simulink library "Gait_Selector"  (R2024a)
settings: Solver=VariableStepAuto  StartTime=0.0  StopTime=10.0  RelTol=1e-3
undefined symbols (not defined in the file): Length_torso, sampleTime, transferFunVal, Width_torso
libraries: simulink_extras x12, stand_still_Gait x1, trot_Gait x1, turn_left_Gait x1, turn_right_Gait x1, walk_back_Gait x1, walk_Gait x1, walk_left_Gait x1, walk_right_Gait x1
(part 1 of 2)
settings Model: Creator=renre  LastModifiedBy=leona

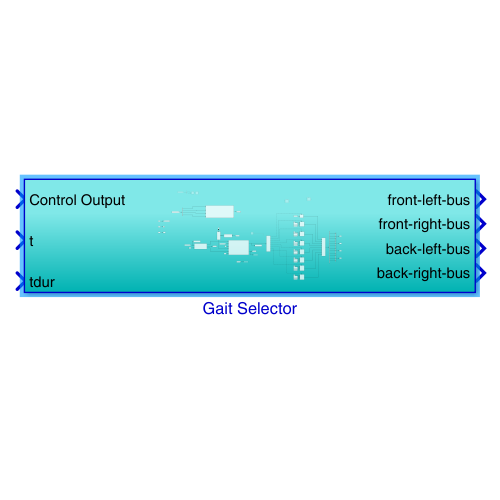
[thumbnail: Simulink's stored preview of the top-level diagram]
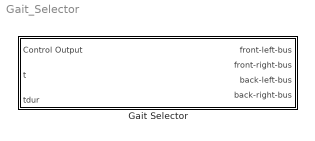
== system Gait_Selector ==
  Gait Selector : Subsystem

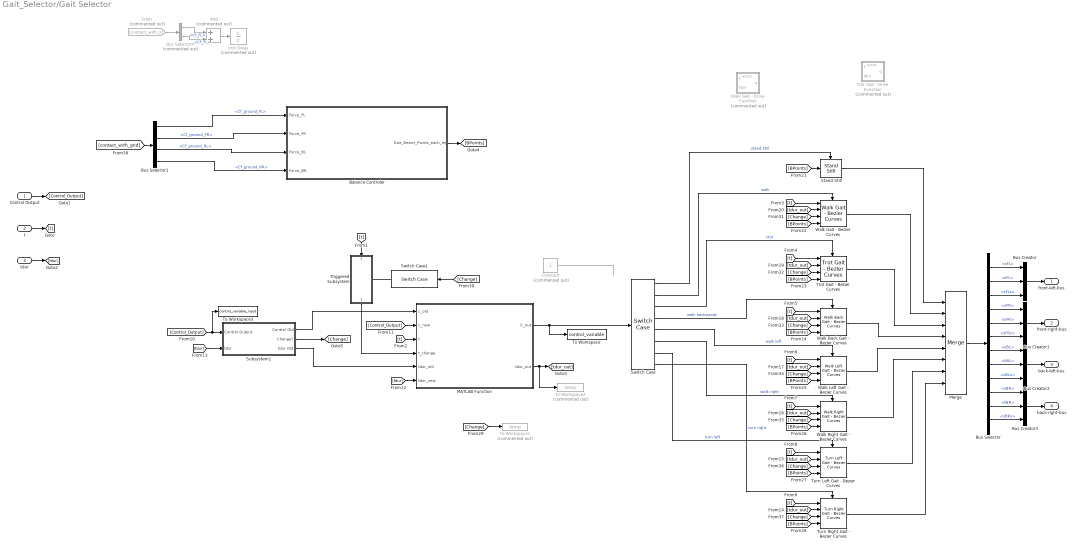
== system Gait_Selector/Gait Selector ==
  Control Output : Inport
  t : Inport  Port=2
  tdur : Inport  Port=3
  Add : Sum  Commented=on
  Balance Controler : Subsystem
  Bus Creator{,1..3} (4 alike) : BusCreator  Inputs=3
  Bus Selector : BusSelector  OutputSignals=sFL,kFL,sFLs,sFR,kFR,sFRs,sBL,kBL,sBLs,sBR,kBR,sBRs
  Bus Selector1 : BusSelector  OutputSignals=Cf_ground_FL,Cf_ground_FR,Cf_ground_RL,Cf_ground_RR
  Bus Selector4 : BusSelector  Commented=on  OutputSignals=Wall.Cf_FL,Slope.Cf_FL
  Constant : Constant  Commented=on
  From : From  Commented=on  GotoTag=contact_with_x  TagVisibility=global
  MATLAB Function : MATLAB Function  TreatAsAtomicUnit=on
  Merge : Merge  Inputs=8
  Stand Still : stand_still_Gait/Stand Still  SystemSampleTime=-1  VariantActivationTime=update diagram  AllowFlexibleInterface=on  Latency=0  AutoFrameSizeCalculation=off
  Subsystem1 : Subsystem
  Switch Case : SwitchCase  CaseConditions={0,1,2,3,4,5,6,7}  ShowDefaultCase=off
  Switch Case1 : SwitchCase  ShowDefaultCase=off
  To Workspace : ToWorkspace  VariableName=control_variable  SaveFormat=Structure With Time  SampleTime=-1
  To Workspace1 : ToWorkspace  Commented=on  VariableName=temp  SaveFormat=Structure With Time  SampleTime=-1
  To Workspace2 : ToWorkspace  Commented=on  VariableName=temp  SaveFormat=Structure With Time  SampleTime=-1
  To Workspace3 : ToWorkspace  VariableName=control_variable_input  SaveFormat=Structure With Time  SampleTime=-1
  Triggered Subsystem : Subsystem  TreatAsAtomicUnit=on
  Trot Gait - Bezier Curves : trot_Gait/Trot Gait - Bezier Curves  SystemSampleTime=-1  VariantActivationTime=update diagram  AllowFlexibleInterface=on  Latency=0  AutoFrameSizeCalculation=off
  Trot Gait - Drive Function : Subsystem  Commented=on  mask{uMin=30-20, uMax=30+10, lMin=-50, lMax=-35}
      mask prompts: uMin "Min Angle Hip"; uMax "Max Angle Hip"; lMin "Min Angle Knee"; lMax "Max Angle Knee"
  Turn Left Gait - Bezier Curves : turn_left_Gait/Turn Left Gait - Bezier Curves  SystemSampleTime=-1  VariantActivationTime=update diagram  AllowFlexibleInterface=on  Latency=0  AutoFrameSizeCalculation=off
  Turn Right Gait - Bezier Curves : turn_right_Gait/Turn Right Gait - Bezier Curves  SystemSampleTime=-1  VariantActivationTime=update diagram  AllowFlexibleInterface=on  Latency=0  AutoFrameSizeCalculation=off
  Unit Delay : UnitDelay  Commented=on  SampleTime=-1  HasFrameUpgradeWarning=on
  Walk Back Gait - Bezier Curves : walk_back_Gait/Walk Back Gait - Bezier Curves  SystemSampleTime=-1  VariantActivationTime=update diagram  AllowFlexibleInterface=on  Latency=0  AutoFrameSizeCalculation=off
  Walk Gait - Bezier Curves : walk_Gait/Walk Gait - Bezier Curves  SystemSampleTime=-1  VariantActivationTime=update diagram  AllowFlexibleInterface=on  Latency=0  AutoFrameSizeCalculation=off
  Walk Gait - Drive Function : Subsystem  Commented=on  mask{uMin=30-20, uMax=30+10, lMin=-50, lMax=-35}
      mask prompts: uMin "Min Angle Hip"; uMax "Max Angle Hip"; lMin "Min Angle Knee"; lMax "Max Angle Knee"
  Walk Left Gait - Bezier Curves : walk_left_Gait/Walk Left Gait - Bezier Curves  SystemSampleTime=-1  VariantActivationTime=update diagram  AllowFlexibleInterface=on  Latency=0  AutoFrameSizeCalculation=off
  Walk Right Gait - Bezier Curves : walk_right_Gait/Walk Right Gait - Bezier Curves  SystemSampleTime=-1  VariantActivationTime=update diagram  AllowFlexibleInterface=on  Latency=0  AutoFrameSizeCalculation=off
  front-left-bus : Outport
  front-right-bus : Outport  Port=2
  back-left-bus : Outport  Port=3
  back-right-bus : Outport  Port=4
  wires:
  Control Output/1 -> [Control_Output]
  t/1 -> [t]
  Bus Creator/1 -> front-left-bus/1
  Bus Creator1/1 -> front-right-bus/1
  Bus Creator2/1 -> back-left-bus/1
  Bus Creator3/1 -> back-right-bus/1
  Switch Case/2 -> Walk Gait - Bezier Curves/Action  "walk"
  Switch Case/3 -> Trot Gait - Bezier Curves/Action  "trot"
  Switch Case/5 -> Walk Left Gait - Bezier Curves/Action  "walk left"
  Switch Case/6 -> Walk Right Gait - Bezier Curves/Action  "walk right"
  Switch Case/7 -> Turn Left Gait - Bezier Curves/Action  "turn left"
  Switch Case/8 -> Turn Right Gait - Bezier Curves/Action  "turn right"
  MATLAB Function/2(tdur_out) -> To Workspace2/1, [tdur_out]
  Merge/1 -> Bus Selector/1
  Walk Gait - Bezier Curves/1 -> Merge/2
  Bus Selector/1 -> Bus Creator/1  "<sFL>"
  Bus Selector/2 -> Bus Creator/2  "<kFL>"
  Bus Selector/6 -> Bus Creator1/3  "<sFRs>"
  Bus Selector/5 -> Bus Creator1/2  "<kFR>"
  Bus Selector/7 -> Bus Creator2/1  "<sBL>"
  Bus Selector/8 -> Bus Creator2/2  "<kBL>"
  Bus Selector/12 -> Bus Creator3/3  "<sBRs>"
  Trot Gait - Bezier Curves/1 -> Merge/3
  Bus Selector/11 -> Bus Creator3/2  "<kBR>"
  Walk Left Gait - Bezier Curves/1 -> Merge/5
  Bus Selector/3 -> Bus Creator/3  "<sFLs>"
  Bus Selector/4 -> Bus Creator1/1  "<sFR>"
  Bus Selector/10 -> Bus Creator3/1  "<sBR>"
  Bus Selector/9 -> Bus Creator2/3  "<sBLs>"
  Walk Right Gait - Bezier Curves/1 -> Merge/6
  Turn Left Gait - Bezier Curves/1 -> Merge/7
  Turn Right Gait - Bezier Curves/1 -> Merge/8
  Switch Case/4 -> Walk Back Gait - Bezier Curves/Action  "walk backwards"
  Walk Back Gait - Bezier Curves/1 -> Merge/4
  Stand Still/1 -> Merge/1
  Switch Case/1 -> Stand Still/Action  "stand still"
  Subsystem1/2(Change?) -> [Change]
  MATLAB Function/1(C_out) -> Switch Case/1, To Workspace/1
  Subsystem1/1(Control Old) -> MATLAB Function/1(c_old)
  tdur/1 -> [tdur]
  Subsystem1/3(tdur Old) -> MATLAB Function/5(tdur_old)
  Triggered Subsystem/1(activationTime) -> MATLAB Function/4(t_change)
  Switch Case1/1 -> Triggered Subsystem/Action
  Constant/1 -> ?
  Balance Controler/1(Gait_Bezier_Points_each_leg) -> [BPoints]
  Add/1 -> Unit Delay/1
  From/1 -> Bus Selector4/1
  Bus Selector4/1 -> Add/1  "<Cf_FL>"
  Bus Selector4/2 -> Add/2  "<Cf_FL>"
  [t] -> Triggered Subsystem/1(t)
  [t] -> MATLAB Function/3(t)
  [t] -> Walk Gait - Bezier Curves/1
  [t] -> Trot Gait - Bezier Curves/1
  [t] -> Walk Back Gait - Bezier Curves/1
  [t] -> Walk Left Gait - Bezier Curves/1
  [t] -> Walk Right Gait - Bezier Curves/1
  [t] -> Turn Left Gait - Bezier Curves/1
  [t] -> Turn Right Gait - Bezier Curves/1
  [Control_Output] -> To Workspace3/1, Subsystem1/1(Control Output)
  [Control_Output] -> MATLAB Function/2(c_new)
  [tdur] -> Subsystem1/2(tdur)
  [tdur] -> MATLAB Function/6(tdur_new)
  [tdur_out] -> Turn Right Gait - Bezier Curves/2
  [tdur_out] -> Turn Left Gait - Bezier Curves/2
  [tdur_out] -> Walk Right Gait - Bezier Curves/2
  [tdur_out] -> Walk Left Gait - Bezier Curves/2
  [tdur_out] -> Walk Back Gait - Bezier Curves/2
  [tdur_out] -> Trot Gait - Bezier Curves/2
  [tdur_out] -> Walk Gait - Bezier Curves/2
  [BPoints] -> Stand Still/1
  [BPoints] -> Walk Gait - Bezier Curves/4
  [BPoints] -> Trot Gait - Bezier Curves/4
  [BPoints] -> Walk Back Gait - Bezier Curves/4
  [BPoints] -> Walk Left Gait - Bezier Curves/4
  [BPoints] -> Walk Right Gait - Bezier Curves/4
  [BPoints] -> Turn Left Gait - Bezier Curves/4
  [BPoints] -> Turn Right Gait - Bezier Curves/4
  [Change] -> To Workspace1/1
  [Change] -> Switch Case1/1
  [Change] -> Walk Gait - Bezier Curves/3
  [Change] -> Trot Gait - Bezier Curves/3
  [Change] -> Walk Back Gait - Bezier Curves/3
  [Change] -> Walk Left Gait - Bezier Curves/3
  [Change] -> Walk Right Gait - Bezier Curves/3
  [Change] -> Turn Left Gait - Bezier Curves/3
  [Change] -> Turn Right Gait - Bezier Curves/3
  [contact_with_grid] -> Bus Selector1/1
  Bus Selector1/3 -> Balance Controler/3(Force_BL)  "<Cf_ground_RL>"
  Bus Selector1/4 -> Balance Controler/4(Force_BR)  "<Cf_ground_RR>"
  Bus Selector1/1 -> Balance Controler/1(Force_FL)  "<Cf_ground_FL>"
  Bus Selector1/2 -> Balance Controler/2(Force_FR)  "<Cf_ground_FR>"

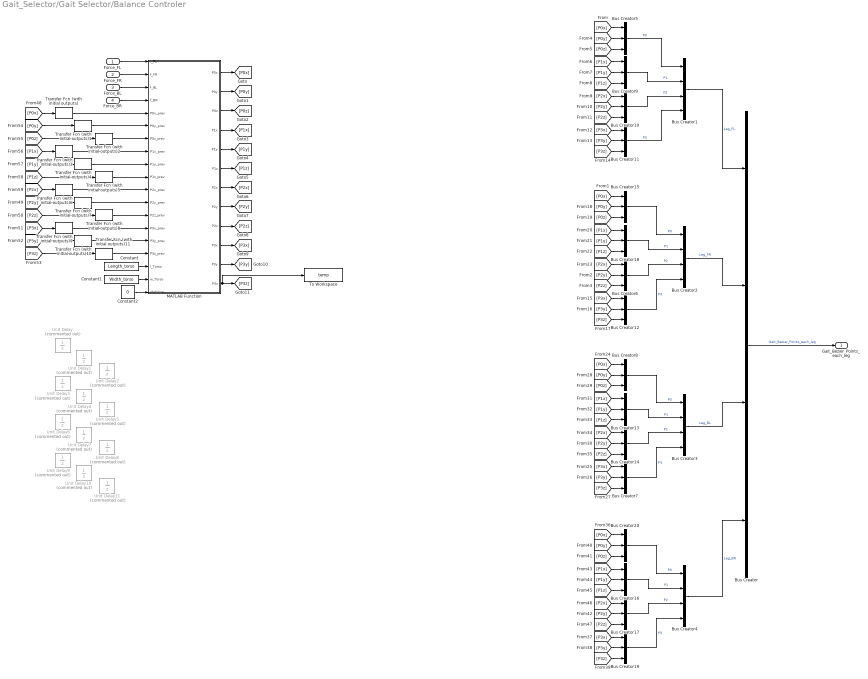
== system Gait_Selector/Gait Selector/Balance Controler ==
  Force_FL : Inport
  Force_FR : Inport  Port=2
  Force_BL : Inport  Port=3
  Force_BR : Inport  Port=4
  Bus Creator{,1..4} (5 alike) : BusCreator  Inputs=4
  Bus Creator{5..20} (16 alike) : BusCreator  Inputs=3
  Constant : Constant  Value=Length_torso
  Constant1 : Constant  Value=Width_torso
  Constant2 : Constant  Value=0
  MATLAB Function : MATLAB Function  TreatAsAtomicUnit=on
  To Workspace : ToWorkspace  VariableName=temp  SaveFormat=Structure With Time  SampleTime=-1
  Transfer Fcn (with initial outputs) : simulink_extras/Additional Linear/Transfer Fcn (with initial outputs)  N=[1]  D=transferFunVal  Y0=-0.02  U0=0
  Transfer Fcn (with initial outputs)1 : simulink_extras/Additional Linear/Transfer Fcn (with initial outputs)  N=[1]  D=transferFunVal  Y0=-0.02  U0=0
  Transfer Fcn (with initial outputs)10 : simulink_extras/Additional Linear/Transfer Fcn (with initial outputs)  N=[1]  D=transferFunVal  Y0=0.02  U0=0
  Transfer Fcn (with initial outputs)11 : simulink_extras/Additional Linear/Transfer Fcn (with initial outputs)  N=[1]  D=transferFunVal  Y0=-0.08  U0=0
  Transfer Fcn (with initial outputs)2 : simulink_extras/Additional Linear/Transfer Fcn (with initial outputs)  N=[1]  D=transferFunVal  Y0=-0.08  U0=0
  Transfer Fcn (with initial outputs)3 : simulink_extras/Additional Linear/Transfer Fcn (with initial outputs)  N=[1]  D=transferFunVal  Y0=-0.035  U0=0
  Transfer Fcn (with initial outputs)4 : simulink_extras/Additional Linear/Transfer Fcn (with initial outputs)  N=[1]  D=transferFunVal  Y0=-0.035  U0=0
  Transfer Fcn (with initial outputs)5 : simulink_extras/Additional Linear/Transfer Fcn (with initial outputs)  N=[1]  D=transferFunVal  Y0=-0.075  U0=0
  Transfer Fcn (with initial outputs)6 : simulink_extras/Additional Linear/Transfer Fcn (with initial outputs)  N=[1]  D=transferFunVal  Y0=0.01  U0=0
  Transfer Fcn (with initial outputs)7 : simulink_extras/Additional Linear/Transfer Fcn (with initial outputs)  N=[1]  D=transferFunVal  Y0=0.01  U0=0
  Transfer Fcn (with initial outputs)8 : simulink_extras/Additional Linear/Transfer Fcn (with initial outputs)  N=[1]  D=transferFunVal  Y0=-0.075  U0=0
  Transfer Fcn (with initial outputs)9 : simulink_extras/Additional Linear/Transfer Fcn (with initial outputs)  N=[1]  D=transferFunVal  Y0=0.02  U0=0
  Unit Delay : UnitDelay  Commented=on  InitialCondition=-0.02  SampleTime=sampleTime  HasFrameUpgradeWarning=on
  Unit Delay1 : UnitDelay  Commented=on  InitialCondition=-0.02  SampleTime=sampleTime  HasFrameUpgradeWarning=on
  Unit Delay10 : UnitDelay  Commented=on  InitialCondition=0.02  SampleTime=sampleTime  HasFrameUpgradeWarning=on
  Unit Delay11 : UnitDelay  Commented=on  InitialCondition=-0.08  SampleTime=sampleTime  HasFrameUpgradeWarning=on
  Unit Delay2 : UnitDelay  Commented=on  InitialCondition=-0.08  SampleTime=sampleTime  HasFrameUpgradeWarning=on
  Unit Delay3 : UnitDelay  Commented=on  InitialCondition=-0.035  SampleTime=sampleTime  HasFrameUpgradeWarning=on
  Unit Delay4 : UnitDelay  Commented=on  InitialCondition=-0.035  SampleTime=sampleTime  HasFrameUpgradeWarning=on
  Unit Delay5 : UnitDelay  Commented=on  InitialCondition=-0.06  SampleTime=sampleTime  HasFrameUpgradeWarning=on
  Unit Delay6 : UnitDelay  Commented=on  InitialCondition=0.01  SampleTime=sampleTime  HasFrameUpgradeWarning=on
  Unit Delay7 : UnitDelay  Commented=on  InitialCondition=0.01  SampleTime=sampleTime  HasFrameUpgradeWarning=on
  Unit Delay8 : UnitDelay  Commented=on  InitialCondition=-0.075  SampleTime=sampleTime  HasFrameUpgradeWarning=on
  Unit Delay9 : UnitDelay  Commented=on  InitialCondition=0.02  SampleTime=sampleTime  HasFrameUpgradeWarning=on
  Gait_Bezier_Points_each_leg : Outport
  wires:
  Bus Creator1/1 -> Bus Creator/1  "Leg_FL"
  Bus Creator2/1 -> Bus Creator/2  "Leg_FR"
  Bus Creator3/1 -> Bus Creator/3  "Leg_BL"
  Bus Creator4/1 -> Bus Creator/4  "Leg_BR"
  Bus Creator/1 -> Gait_Bezier_Points_each_leg/1  "Gait_Bezier_Points_each_leg"
  Bus Creator5/1 -> Bus Creator1/1  "P0"
  Bus Creator9/1 -> Bus Creator1/2  "P1"
  Bus Creator10/1 -> Bus Creator1/3  "P2"
  Bus Creator11/1 -> Bus Creator1/4  "P3"
  MATLAB Function/1(P0x) -> [P0x]
  Force_FL/1 -> MATLAB Function/1(f_FL)
  Force_FR/1 -> MATLAB Function/2(f_FR)
  Force_BL/1 -> MATLAB Function/3(f_BL)
  Force_BR/1 -> MATLAB Function/4(f_BR)
  [P0x] -> Transfer Fcn (with initial outputs)/1
  [P0z] -> Transfer Fcn (with initial outputs)2/1
  [P0y] -> Transfer Fcn (with initial outputs)1/1
  [P1y] -> Transfer Fcn (with initial outputs)4/1
  [P1x] -> Transfer Fcn (with initial outputs)3/1
  [P1z] -> Transfer Fcn (with initial outputs)5/1
  Constant/1 -> MATLAB Function/17(l_Torso)
  Constant1/1 -> MATLAB Function/18(w_Torso)
  [P0x] -> Bus Creator5/1
  [P0y] -> Bus Creator5/2
  [P0z] -> Bus Creator5/3
  MATLAB Function/2(P0y) -> [P0y]
  MATLAB Function/3(P0z) -> [P0z]
  MATLAB Function/6(P1z) -> [P1z]
  MATLAB Function/5(P1y) -> [P1y]
  MATLAB Function/4(P1x) -> [P1x]
  MATLAB Function/10(P3x) -> [P3x]
  MATLAB Function/11(P3y) -> [P3y]
  MATLAB Function/12(P3z) -> To Workspace/1, [P3z]
  MATLAB Function/9(P2z) -> [P2z]
  MATLAB Function/8(P2y) -> [P2y]
  MATLAB Function/7(P2x) -> [P2x]
  [P1y] -> Bus Creator9/2
  [P1x] -> Bus Creator9/1
  [P1z] -> Bus Creator9/3
  [P3z] -> Bus Creator11/3
  [P3x] -> Bus Creator11/1
  [P3y] -> Bus Creator11/2
  [P2z] -> Bus Creator10/3
  [P2y] -> Bus Creator10/2
  [P2x] -> Bus Creator10/1
  [P2x] -> Bus Creator6/1
  [P2y] -> Bus Creator6/2
  [P2z] -> Bus Creator6/3
  [P3y] -> Bus Creator12/2
  [P3x] -> Bus Creator12/1
  [P3z] -> Bus Creator12/3
  [P1z] -> Bus Creator18/3
  [P1x] -> Bus Creator18/1
  [P1y] -> Bus Creator18/2
  [P0z] -> Bus Creator15/3
  [P0y] -> Bus Creator15/2
  [P0x] -> Bus Creator15/1
  Bus Creator12/1 -> Bus Creator2/4  "P3"
  Bus Creator6/1 -> Bus Creator2/3  "P2"
  Bus Creator18/1 -> Bus Creator2/2  "P1"
  Bus Creator15/1 -> Bus Creator2/1  "P0"
  Bus Creator8/1 -> Bus Creator3/1  "P0"
  Bus Creator13/1 -> Bus Creator3/2  "P1"
  Bus Creator14/1 -> Bus Creator3/3  "P2"
  Bus Creator7/1 -> Bus Creator3/4  "P3"
  [P0x] -> Bus Creator8/1
  [P0y] -> Bus Creator8/2
  [P0z] -> Bus Creator8/3
  [P1y] -> Bus Creator13/2
  [P1x] -> Bus Creator13/1
  [P1z] -> Bus Creator13/3
  [P3z] -> Bus Creator7/3
  [P3x] -> Bus Creator7/1
  [P3y] -> Bus Creator7/2
  [P2z] -> Bus Creator14/3
  [P2y] -> Bus Creator14/2
  [P2x] -> Bus Creator14/1
  [P2x] -> Bus Creator17/1
  [P2y] -> Bus Creator17/2
  [P2z] -> Bus Creator17/3
  [P3y] -> Bus Creator19/2
  [P3x] -> Bus Creator19/1
  [P3z] -> Bus Creator19/3
  [P1z] -> Bus Creator16/3
  [P1x] -> Bus Creator16/1
  [P1y] -> Bus Creator16/2
  [P0z] -> Bus Creator20/3
  [P0y] -> Bus Creator20/2
  [P0x] -> Bus Creator20/1
  Bus Creator19/1 -> Bus Creator4/4  "P3"
  Bus Creator17/1 -> Bus Creator4/3  "P2"
  Bus Creator16/1 -> Bus Creator4/2  "P1"
  Bus Creator20/1 -> Bus Creator4/1  "P0"
  Constant2/1 -> MATLAB Function/19(stabilize)
  [P2y] -> Transfer Fcn (with initial outputs)7/1
  [P2z] -> Transfer Fcn (with initial outputs)8/1
  [P2x] -> Transfer Fcn (with initial outputs)6/1
  [P3x] -> Transfer Fcn (with initial outputs)9/1
  [P3z] -> Transfer Fcn (with initial outputs)11/1
  [P3y] -> Transfer Fcn (with initial outputs)10/1
  Transfer Fcn (with initial outputs)1/1 -> MATLAB Function/6(P0y_prev)
  Transfer Fcn (with initial outputs)11/1 -> MATLAB Function/16(P3z_prev)
  Transfer Fcn (with initial outputs)2/1 -> MATLAB Function/7(P0z_prev)
  Transfer Fcn (with initial outputs)10/1 -> MATLAB Function/15(P3y_prev)
  Transfer Fcn (with initial outputs)/1 -> MATLAB Function/5(P0x_prev)
  Transfer Fcn (with initial outputs)6/1 -> MATLAB Function/11(P2x_prev)
  Transfer Fcn (with initial outputs)4/1 -> MATLAB Function/9(P1y_prev)
  Transfer Fcn (with initial outputs)7/1 -> MATLAB Function/12(P2y_prev)
  Transfer Fcn (with initial outputs)3/1 -> MATLAB Function/8(P1x_prev)
  Transfer Fcn (with initial outputs)5/1 -> MATLAB Function/10(P1z_prev)
  Transfer Fcn (with initial outputs)9/1 -> MATLAB Function/14(P3x_prev)
  Transfer Fcn (with initial outputs)8/1 -> MATLAB Function/13(P2z_prev)

== system Gait_Selector/Gait Selector/Subsystem1 ==
  Control Output : Inport
  tdur : Inport  Port=2
  Data Type Conversion : DataTypeConversion  OutDataTypeStr=double  SaturateOnIntegerOverflow=off  RndMeth=Floor
  Memory{,1..3} (4 alike) : Memory
  OR : Logic  Operator=OR  IconShape=distinctive  AllPortsSameDT=off  OutDataTypeStr=boolean
  Relational Operator : RelationalOperator  Operator=~=  OutDataTypeStr=boolean  RndMeth=Simplest  InputSameDT=off
  Relational Operator1 : RelationalOperator  Operator=~=  OutDataTypeStr=boolean  RndMeth=Simplest  InputSameDT=off
  Switch : Switch  Criteria=u2 > Threshold  SaturateOnIntegerOverflow=off  InputSameDT=off
  Switch1 : Switch  Criteria=u2 > Threshold  SaturateOnIntegerOverflow=off  InputSameDT=off
  Switch2 : Switch  Criteria=u2 ~= 0  SaturateOnIntegerOverflow=off  InputSameDT=off
  Unit Delay : UnitDelay  SampleTime=-1  HasFrameUpgradeWarning=on
  Unit Delay1 : UnitDelay  SampleTime=-1  HasFrameUpgradeWarning=on
  Control Old : Outport
  Change? : Outport  Port=2
  tdur Old : Outport  Port=3
  wires:
  Unit Delay/1 -> Memory/1, Relational Operator/1
  Relational Operator/1 -> Switch/2, OR/1
  Control Output/1 -> Relational Operator/2, Unit Delay/1
  Unit Delay1/1 -> Memory1/1, Relational Operator1/1
  Relational Operator1/1 -> Switch1/2, OR/2
  OR/1 -> Data Type Conversion/1
  Switch/1 -> Memory2/1, Control Old/1
  Switch1/1 -> Switch2/1, Switch2/2, Memory3/1
  Memory1/1 -> Switch1/1
  Memory/1 -> Switch/1
  Data Type Conversion/1 -> Change?/1
  Switch2/1 -> tdur Old/1
  tdur/1 -> Switch2/3, Relational Operator1/2, Unit Delay1/1
  Memory2/1 -> Switch/3
  Memory3/1 -> Switch1/3

== system Gait_Selector/Gait Selector/Triggered Subsystem ==
  t : Inport
  Action Port : ActionPort  InitializeStates=reset
  MATLAB Function : MATLAB Function  TreatAsAtomicUnit=on
  activationTime : Outport
  wires:
  MATLAB Function/1(activationTime) -> activationTime/1
  t/1 -> MATLAB Function/1(u)

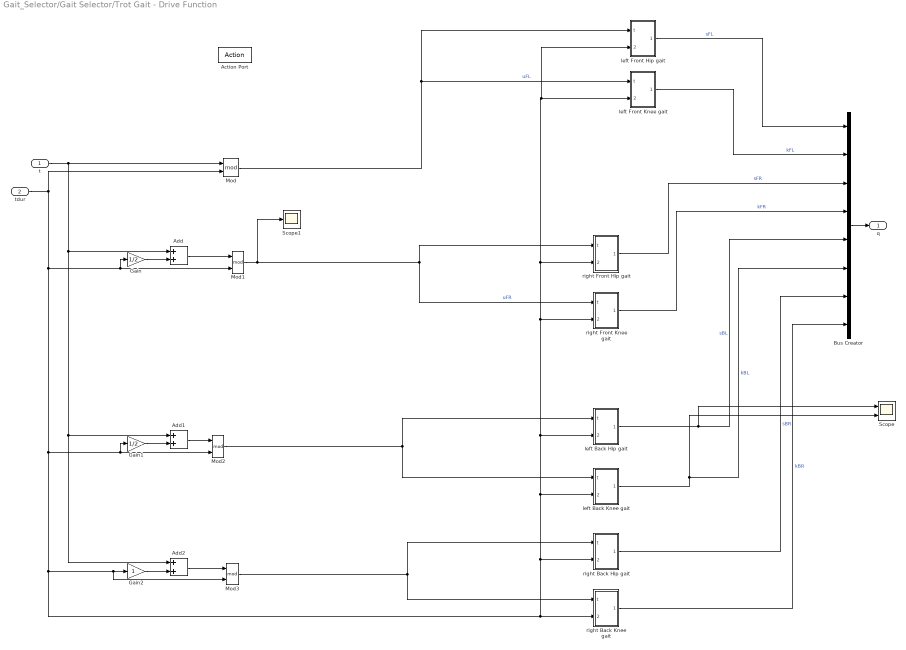
== system Gait_Selector/Gait Selector/Trot Gait - Drive Function ==
  t : Inport
  tdur : Inport  Port=2
  Action Port : ActionPort
  Add : Sum
  Add1 : Sum
  Add2 : Sum
  Bus Creator : BusCreator  Inputs=8
  Gain : Gain  Gain=1/2
  Gain1 : Gain  Gain=1/2
  Gain2 : Gain
  Mod{,1..3} (4 alike) : Math  Operator=mod
  Scope : Scope  NumInputPorts=2
  Scope1 : Scope
  left Back Hip gait : Subsystem
  left Back Knee gait : Subsystem
  left Front Hip gait : Subsystem
  left Front Knee gait : Subsystem
  right Back Hip gait : Subsystem
  right Back Knee gait : Subsystem
  right Front Hip gait : Subsystem
  right Front Knee gait : Subsystem
  q : Outport
  wires:
  Bus Creator/1 -> q/1
  left Front Hip gait/1(Out1) -> Bus Creator/1  "sFL"
  right Front Hip gait/1(Out1) -> Bus Creator/3  "sFR"
  left Front Knee gait/1(Out1) -> Bus Creator/2  "kFL"
  right Front Knee gait/1(Out1) -> Bus Creator/4  "kFR"
  Mod/1 -> left Front Hip gait/1(t), left Front Knee gait/1(t)  "uFL"
  Mod1/1 -> Scope1/1, right Front Hip gait/1(t), right Front Knee gait/1(t)  "uFR"
  left Back Knee gait/1(Out1) -> Scope/2, Bus Creator/6  "kBL"
  left Back Hip gait/1(Out1) -> Scope/1, Bus Creator/5  "sBL"
  right Back Knee gait/1(Out1) -> Bus Creator/8  "kBR"
  right Back Hip gait/1(Out1) -> Bus Creator/7  "sBR"
  Mod2/1 -> left Back Hip gait/1(t), left Back Knee gait/1(t)
  Mod3/1 -> right Back Knee gait/1(t), right Back Hip gait/1(t)
  t/1 -> Mod/1, Add2/1, Add1/1, Add/1
  Gain2/1 -> Add2/2
  tdur/1 -> Mod/2, left Back Knee gait/2(tdur), left Back Hip gait/2(tdur), right Front Knee gait/2(tdur), right Front Hip gait/2(tdur), left Front Hip gait/2(tdur), left Front Knee gait/2(tdur), right Back Hip gait/2(tdur), right Back Knee gait/2(tdur), Gain2/1, Mod3/2, Mod2/2, Gain1/1, Gain/1, Mod1/2
  Add1/1 -> Mod2/1
  Add/1 -> Mod1/1
  Gain/1 -> Add/2
  Gain1/1 -> Add1/2
  Add2/1 -> Mod3/1

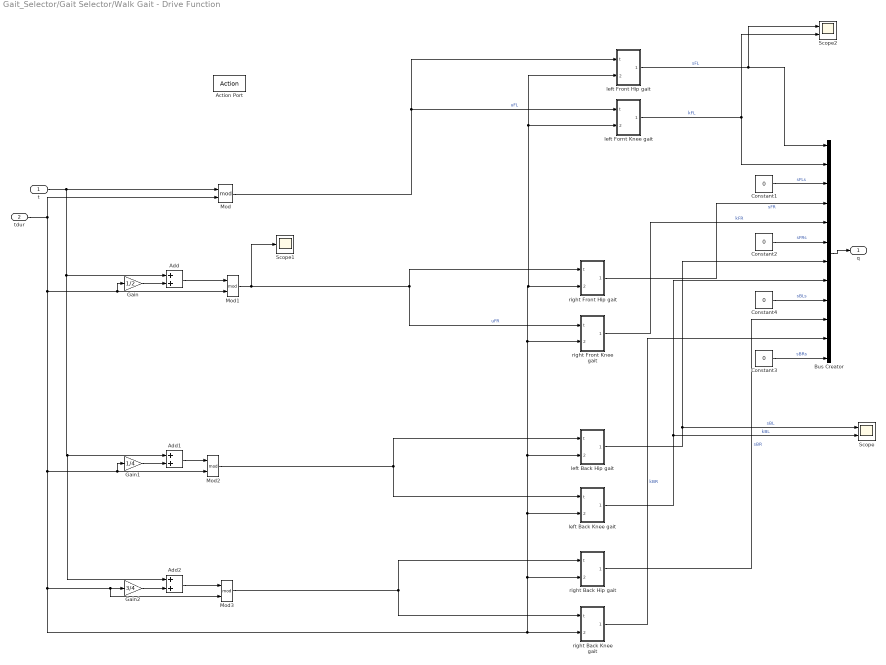
== system Gait_Selector/Gait Selector/Walk Gait - Drive Function ==
  t : Inport
  tdur : Inport  Port=2
  Action Port : ActionPort  InitializeStates=reset
  Add : Sum
  Add1 : Sum
  Add2 : Sum
  Bus Creator : BusCreator  Inputs=12
  Constant{1..4} (4 alike) : Constant  Value=0
  Gain : Gain  Gain=1/2
  Gain1 : Gain  Gain=1/4
  Gain2 : Gain  Gain=3/4
  Mod{,1..3} (4 alike) : Math  Operator=mod
  Scope : Scope  NumInputPorts=2
  Scope1 : Scope
  Scope2 : Scope  NumInputPorts=2
  left Back Hip gait : Subsystem
  left Back Knee gait : Subsystem
  left Fornt Knee gait : Subsystem
  left Front Hip gait : Subsystem
  right Back Hip gait : Subsystem
  right Back Knee gait : Subsystem
  right Front Hip gait : Subsystem
  right Front Knee gait : Subsystem
  q : Outport
  wires:
  Bus Creator/1 -> q/1
  left Front Hip gait/1(Out1) -> Scope2/1, Bus Creator/1  "sFL"
  right Front Hip gait/1(Out1) -> Bus Creator/4  "sFR"
  left Fornt Knee gait/1(Out1) -> Scope2/2, Bus Creator/2  "kFL"
  right Front Knee gait/1(Out1) -> Bus Creator/5  "kFR"
  Mod/1 -> left Front Hip gait/1(t), left Fornt Knee gait/1(t)  "uFL"
  Mod1/1 -> Scope1/1, right Front Hip gait/1(t), right Front Knee gait/1(t)  "uFR"
  left Back Knee gait/1(Out1) -> Scope/2, Bus Creator/8  "kBL"
  left Back Hip gait/1(Out1) -> Scope/1, Bus Creator/7  "sBL"
  right Back Knee gait/1(Out1) -> Bus Creator/11  "kBR"
  right Back Hip gait/1(Out1) -> Bus Creator/10  "sBR"
  Mod2/1 -> left Back Hip gait/1(t), left Back Knee gait/1(t)
  Mod3/1 -> right Back Knee gait/1(t), right Back Hip gait/1(t)
  t/1 -> Mod/1, Add2/1, Add1/1, Add/1
  Gain2/1 -> Add2/2
  tdur/1 -> Mod/2, left Back Knee gait/2(tdur), left Back Hip gait/2(tdur), right Front Knee gait/2(tdur), right Front Hip gait/2(tdur), left Front Hip gait/2(tdur), left Fornt Knee gait/2(tdur), right Back Hip gait/2(tdur), right Back Knee gait/2(tdur), Gain2/1, Mod3/2, Mod2/2, Gain1/1, Gain/1, Mod1/2
  Add1/1 -> Mod2/1
  Add/1 -> Mod1/1
  Gain/1 -> Add/2
  Gain1/1 -> Add1/2
  Add2/1 -> Mod3/1
  Constant1/1 -> Bus Creator/3  "sFLs"
  Constant3/1 -> Bus Creator/12  "sBRs"
  Constant4/1 -> Bus Creator/9  "sBLs"
  Constant2/1 -> Bus Creator/6  "sFRs"

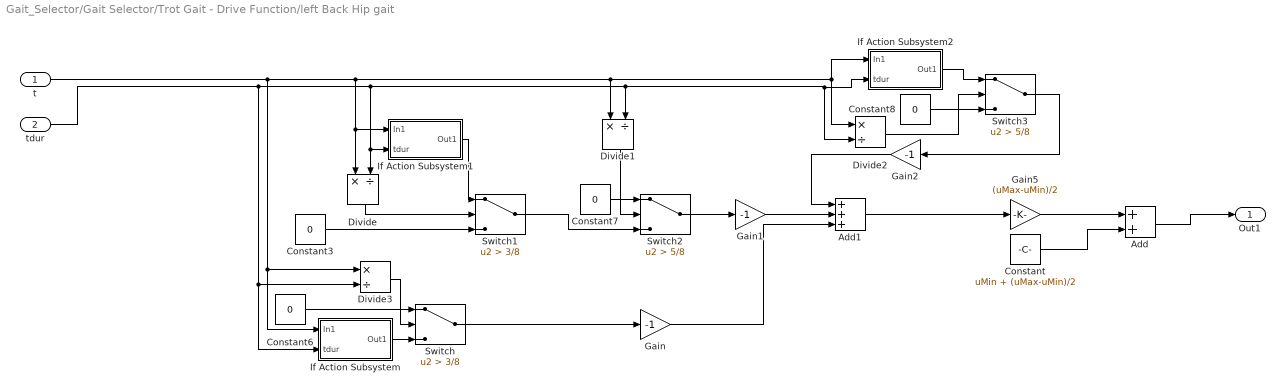
== system Gait_Selector/Gait Selector/Trot Gait - Drive Function/left Back Hip gait ==
  t : Inport
  tdur : Inport  Port=2
  Add : Sum
  Add1 : Sum  Inputs=+++
  Constant : Constant  Value=uMin + (uMax-uMin)/2
  Constant{3,6..8} (4 alike) : Constant  Value=0
  Divide{,1..3} (4 alike) : Product  Inputs=*/
  Gain : Gain  Gain=-1
  Gain1 : Gain  Gain=-1
  Gain2 : Gain  Gain=-1
  Gain5 : Gain  Gain=(uMax-uMin)/2
  If Action Subsystem : Subsystem  TreatAsAtomicUnit=on
  If Action Subsystem1 : Subsystem  TreatAsAtomicUnit=on
  If Action Subsystem2 : Subsystem  TreatAsAtomicUnit=on
  Switch : Switch  Criteria=u2 > Threshold  Threshold=3/8  SaturateOnIntegerOverflow=off  InputSameDT=off
  Switch1 : Switch  Criteria=u2 > Threshold  Threshold=3/8  SaturateOnIntegerOverflow=off  InputSameDT=off
  Switch2 : Switch  Criteria=u2 > Threshold  Threshold=5/8  SaturateOnIntegerOverflow=off  InputSameDT=off
  Switch3 : Switch  Criteria=u2 > Threshold  Threshold=5/8  SaturateOnIntegerOverflow=off  InputSameDT=off
  Out1 : Outport
  wires:
  If Action Subsystem1/1(Out1) -> Switch1/1
  Constant7/1 -> Switch2/1
  Switch1/1 -> Switch2/3
  t/1 -> If Action Subsystem2/1(In1), Divide2/1, Divide1/1, Divide/1, If Action Subsystem1/1(In1), If Action Subsystem/1(In1), Divide3/1
  Add1/1 -> Gain5/1
  If Action Subsystem2/1(Out1) -> Switch3/1
  Switch/1 -> Gain/1
  If Action Subsystem/1(Out1) -> Switch/3
  Constant3/1 -> Switch1/3
  Constant8/1 -> Switch3/3
  Switch3/1 -> Gain2/1
  Switch2/1 -> Gain1/1
  Constant6/1 -> Switch/1
  Gain5/1 -> Add/1
  Constant/1 -> Add/2
  Add/1 -> Out1/1
  Gain/1 -> Add1/3
  Gain1/1 -> Add1/2
  Gain2/1 -> Add1/1
  tdur/1 -> If Action Subsystem/2(tdur), Divide3/2, Divide/2, If Action Subsystem1/2(tdur), If Action Subsystem2/2(tdur), Divide2/2, Divide1/2
  Divide/1 -> Switch1/2
  Divide1/1 -> Switch2/2
  Divide2/1 -> Switch3/2
  Divide3/1 -> Switch/2

== system Gait_Selector/Gait Selector/Trot Gait - Drive Function/left Back Knee gait ==
  t : Inport
  tdur : Inport  Port=2
  Add : Sum
  Constant : Constant  Value=lMin
  Constant10 : Constant  Value=0
  Constant4 : Constant  Value=0
  Divide : Product  Inputs=*/
  Divide1 : Product  Inputs=*/
  Gain7 : Gain  Gain=-(lMax-lMin)
  If Action Subsystem4 : Subsystem  TreatAsAtomicUnit=on
  Switch5 : Switch  Criteria=u2 > Threshold  Threshold=3/8  SaturateOnIntegerOverflow=off  InputSameDT=off
  Switch6 : Switch  Criteria=u2 > Threshold  Threshold=5/8  SaturateOnIntegerOverflow=off  InputSameDT=off
  Out1 : Outport
  wires:
  If Action Subsystem4/1(Out1) -> Switch5/1
  Switch5/1 -> Switch6/3
  t/1 -> Divide1/1, Divide/1, If Action Subsystem4/1(In1)
  Constant4/1 -> Switch5/3
  Constant10/1 -> Switch6/1
  Switch6/1 -> Gain7/1
  Gain7/1 -> Add/1
  Add/1 -> Out1/1
  Constant/1 -> Add/2
  Divide/1 -> Switch5/2
  tdur/1 -> If Action Subsystem4/2(tdur), Divide1/2, Divide/2
  Divide1/1 -> Switch6/2

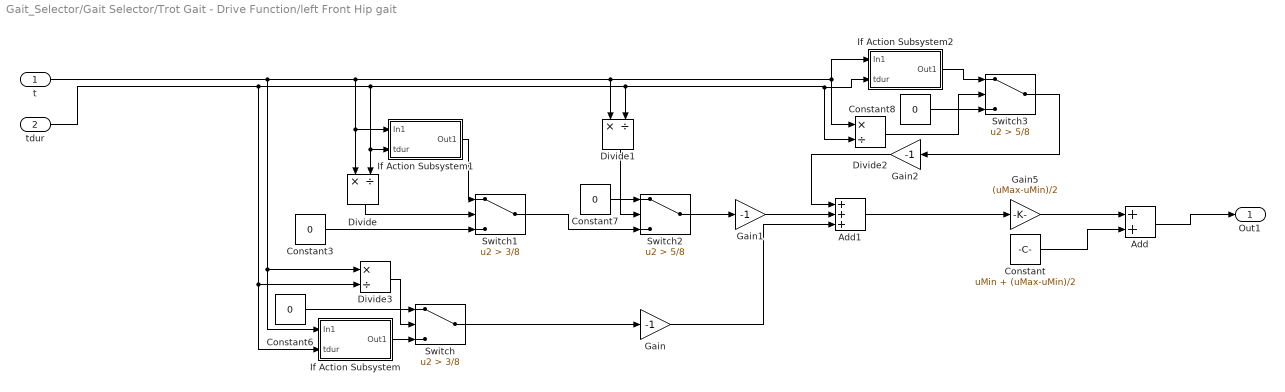
== system Gait_Selector/Gait Selector/Trot Gait - Drive Function/left Front Hip gait ==
  t : Inport
  tdur : Inport  Port=2
  Add : Sum
  Add1 : Sum  Inputs=+++
  Constant : Constant  Value=uMin + (uMax-uMin)/2
  Constant{3,6..8} (4 alike) : Constant  Value=0
  Divide{,1..3} (4 alike) : Product  Inputs=*/
  Gain : Gain  Gain=-1
  Gain1 : Gain  Gain=-1
  Gain2 : Gain  Gain=-1
  Gain5 : Gain  Gain=(uMax-uMin)/2
  If Action Subsystem : Subsystem  TreatAsAtomicUnit=on
  If Action Subsystem1 : Subsystem  TreatAsAtomicUnit=on
  If Action Subsystem2 : Subsystem  TreatAsAtomicUnit=on
  Switch : Switch  Criteria=u2 > Threshold  Threshold=3/8  SaturateOnIntegerOverflow=off  InputSameDT=off
  Switch1 : Switch  Criteria=u2 > Threshold  Threshold=3/8  SaturateOnIntegerOverflow=off  InputSameDT=off
  Switch2 : Switch  Criteria=u2 > Threshold  Threshold=5/8  SaturateOnIntegerOverflow=off  InputSameDT=off
  Switch3 : Switch  Criteria=u2 > Threshold  Threshold=5/8  SaturateOnIntegerOverflow=off  InputSameDT=off
  Out1 : Outport
  wires:
  If Action Subsystem1/1(Out1) -> Switch1/1
  Constant7/1 -> Switch2/1
  Switch1/1 -> Switch2/3
  t/1 -> If Action Subsystem2/1(In1), Divide2/1, Divide1/1, Divide/1, If Action Subsystem1/1(In1), If Action Subsystem/1(In1), Divide3/1
  Add1/1 -> Gain5/1
  If Action Subsystem2/1(Out1) -> Switch3/1
  Switch/1 -> Gain/1
  If Action Subsystem/1(Out1) -> Switch/3
  Constant3/1 -> Switch1/3
  Constant8/1 -> Switch3/3
  Switch3/1 -> Gain2/1
  Switch2/1 -> Gain1/1
  Constant6/1 -> Switch/1
  Gain5/1 -> Add/1
  Constant/1 -> Add/2
  Add/1 -> Out1/1
  Gain/1 -> Add1/3
  Gain1/1 -> Add1/2
  Gain2/1 -> Add1/1
  tdur/1 -> If Action Subsystem/2(tdur), Divide3/2, Divide/2, If Action Subsystem1/2(tdur), If Action Subsystem2/2(tdur), Divide2/2, Divide1/2
  Divide/1 -> Switch1/2
  Divide1/1 -> Switch2/2
  Divide2/1 -> Switch3/2
  Divide3/1 -> Switch/2

== system Gait_Selector/Gait Selector/Trot Gait - Drive Function/left Front Knee gait ==
  t : Inport
  tdur : Inport  Port=2
  Add : Sum
  Constant : Constant  Value=lMin
  Constant10 : Constant  Value=0
  Constant4 : Constant  Value=0
  Divide : Product  Inputs=*/
  Divide1 : Product  Inputs=*/
  Gain7 : Gain  Gain=-(lMax-lMin)
  If Action Subsystem4 : Subsystem  TreatAsAtomicUnit=on
  Switch5 : Switch  Criteria=u2 > Threshold  Threshold=3/8  SaturateOnIntegerOverflow=off  InputSameDT=off
  Switch6 : Switch  Criteria=u2 > Threshold  Threshold=5/8  SaturateOnIntegerOverflow=off  InputSameDT=off
  Out1 : Outport
  wires:
  If Action Subsystem4/1(Out1) -> Switch5/1
  Switch5/1 -> Switch6/3
  t/1 -> Divide1/1, Divide/1, If Action Subsystem4/1(In1)
  Constant4/1 -> Switch5/3
  Constant10/1 -> Switch6/1
  Switch6/1 -> Gain7/1
  Gain7/1 -> Add/1
  Add/1 -> Out1/1
  Constant/1 -> Add/2
  Divide/1 -> Switch5/2
  tdur/1 -> If Action Subsystem4/2(tdur), Divide1/2, Divide/2
  Divide1/1 -> Switch6/2

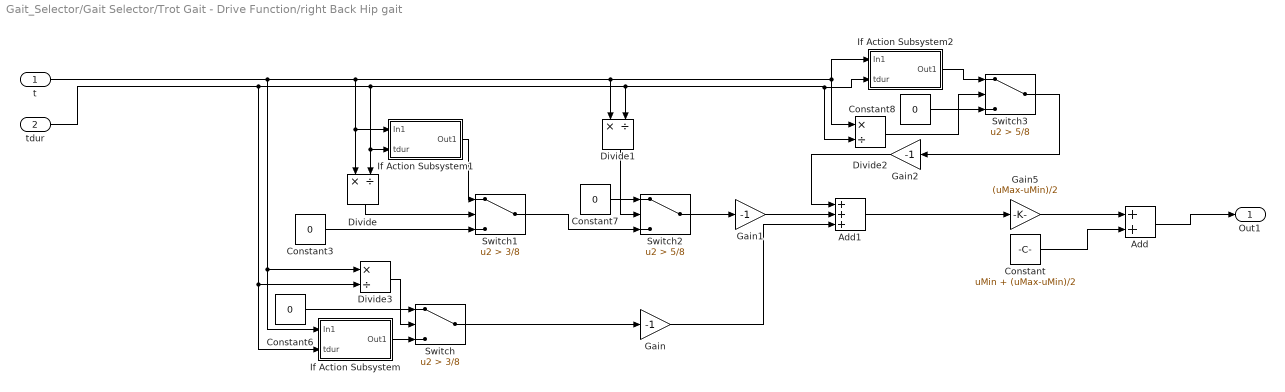
== system Gait_Selector/Gait Selector/Trot Gait - Drive Function/right Back Hip gait ==
  t : Inport
  tdur : Inport  Port=2
  Add : Sum
  Add1 : Sum  Inputs=+++
  Constant : Constant  Value=uMin + (uMax-uMin)/2
  Constant{3,6..8} (4 alike) : Constant  Value=0
  Divide{,1..3} (4 alike) : Product  Inputs=*/
  Gain : Gain  Gain=-1
  Gain1 : Gain  Gain=-1
  Gain2 : Gain  Gain=-1
  Gain5 : Gain  Gain=(uMax-uMin)/2
  If Action Subsystem : Subsystem  TreatAsAtomicUnit=on
  If Action Subsystem1 : Subsystem  TreatAsAtomicUnit=on
  If Action Subsystem2 : Subsystem  TreatAsAtomicUnit=on
  Switch : Switch  Criteria=u2 > Threshold  Threshold=3/8  SaturateOnIntegerOverflow=off  InputSameDT=off
  Switch1 : Switch  Criteria=u2 > Threshold  Threshold=3/8  SaturateOnIntegerOverflow=off  InputSameDT=off
  Switch2 : Switch  Criteria=u2 > Threshold  Threshold=5/8  SaturateOnIntegerOverflow=off  InputSameDT=off
  Switch3 : Switch  Criteria=u2 > Threshold  Threshold=5/8  SaturateOnIntegerOverflow=off  InputSameDT=off
  Out1 : Outport
  wires:
  If Action Subsystem1/1(Out1) -> Switch1/1
  Constant7/1 -> Switch2/1
  Switch1/1 -> Switch2/3
  t/1 -> If Action Subsystem2/1(In1), Divide2/1, Divide1/1, Divide/1, If Action Subsystem1/1(In1), If Action Subsystem/1(In1), Divide3/1
  Add1/1 -> Gain5/1
  If Action Subsystem2/1(Out1) -> Switch3/1
  Switch/1 -> Gain/1
  If Action Subsystem/1(Out1) -> Switch/3
  Constant3/1 -> Switch1/3
  Constant8/1 -> Switch3/3
  Switch3/1 -> Gain2/1
  Switch2/1 -> Gain1/1
  Constant6/1 -> Switch/1
  Gain5/1 -> Add/1
  Constant/1 -> Add/2
  Add/1 -> Out1/1
  Gain/1 -> Add1/3
  Gain1/1 -> Add1/2
  Gain2/1 -> Add1/1
  tdur/1 -> If Action Subsystem/2(tdur), Divide3/2, Divide/2, If Action Subsystem1/2(tdur), If Action Subsystem2/2(tdur), Divide2/2, Divide1/2
  Divide/1 -> Switch1/2
  Divide1/1 -> Switch2/2
  Divide2/1 -> Switch3/2
  Divide3/1 -> Switch/2

== system Gait_Selector/Gait Selector/Trot Gait - Drive Function/right Back Knee gait ==
  t : Inport
  tdur : Inport  Port=2
  Add : Sum
  Constant : Constant  Value=lMin
  Constant10 : Constant  Value=0
  Constant4 : Constant  Value=0
  Divide : Product  Inputs=*/
  Divide1 : Product  Inputs=*/
  Gain7 : Gain  Gain=-(lMax-lMin)
  If Action Subsystem4 : Subsystem  TreatAsAtomicUnit=on
  Switch5 : Switch  Criteria=u2 > Threshold  Threshold=3/8  SaturateOnIntegerOverflow=off  InputSameDT=off
  Switch6 : Switch  Criteria=u2 > Threshold  Threshold=5/8  SaturateOnIntegerOverflow=off  InputSameDT=off
  Out1 : Outport
  wires:
  If Action Subsystem4/1(Out1) -> Switch5/1
  Switch5/1 -> Switch6/3
  t/1 -> Divide1/1, Divide/1, If Action Subsystem4/1(In1)
  Constant4/1 -> Switch5/3
  Constant10/1 -> Switch6/1
  Switch6/1 -> Gain7/1
  Gain7/1 -> Add/1
  Add/1 -> Out1/1
  Constant/1 -> Add/2
  Divide/1 -> Switch5/2
  tdur/1 -> If Action Subsystem4/2(tdur), Divide1/2, Divide/2
  Divide1/1 -> Switch6/2

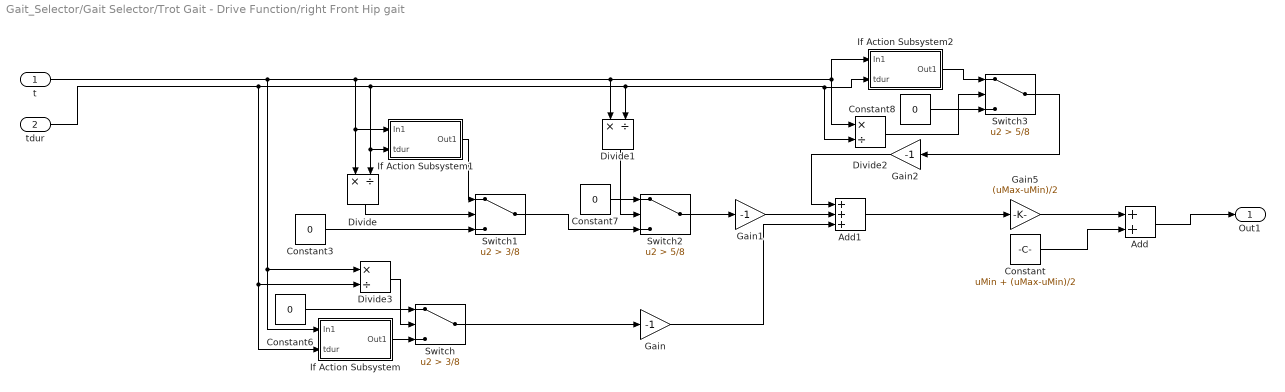
== system Gait_Selector/Gait Selector/Trot Gait - Drive Function/right Front Hip gait ==
  t : Inport
  tdur : Inport  Port=2
  Add : Sum
  Add1 : Sum  Inputs=+++
  Constant : Constant  Value=uMin + (uMax-uMin)/2
  Constant{3,6..8} (4 alike) : Constant  Value=0
  Divide{,1..3} (4 alike) : Product  Inputs=*/
  Gain : Gain  Gain=-1
  Gain1 : Gain  Gain=-1
  Gain2 : Gain  Gain=-1
  Gain5 : Gain  Gain=(uMax-uMin)/2
  If Action Subsystem : Subsystem  TreatAsAtomicUnit=on
  If Action Subsystem1 : Subsystem  TreatAsAtomicUnit=on
  If Action Subsystem2 : Subsystem  TreatAsAtomicUnit=on
  Switch : Switch  Criteria=u2 > Threshold  Threshold=3/8  SaturateOnIntegerOverflow=off  InputSameDT=off
  Switch1 : Switch  Criteria=u2 > Threshold  Threshold=3/8  SaturateOnIntegerOverflow=off  InputSameDT=off
  Switch2 : Switch  Criteria=u2 > Threshold  Threshold=5/8  SaturateOnIntegerOverflow=off  InputSameDT=off
  Switch3 : Switch  Criteria=u2 > Threshold  Threshold=5/8  SaturateOnIntegerOverflow=off  InputSameDT=off
  Out1 : Outport
  wires:
  If Action Subsystem1/1(Out1) -> Switch1/1
  Constant7/1 -> Switch2/1
  Switch1/1 -> Switch2/3
  t/1 -> If Action Subsystem2/1(In1), Divide2/1, Divide1/1, Divide/1, If Action Subsystem1/1(In1), If Action Subsystem/1(In1), Divide3/1
  Add1/1 -> Gain5/1
  If Action Subsystem2/1(Out1) -> Switch3/1
  Switch/1 -> Gain/1
  If Action Subsystem/1(Out1) -> Switch/3
  Constant3/1 -> Switch1/3
  Constant8/1 -> Switch3/3
  Switch3/1 -> Gain2/1
  Switch2/1 -> Gain1/1
  Constant6/1 -> Switch/1
  Gain5/1 -> Add/1
  Constant/1 -> Add/2
  Add/1 -> Out1/1
  Gain/1 -> Add1/3
  Gain1/1 -> Add1/2
  Gain2/1 -> Add1/1
  tdur/1 -> If Action Subsystem/2(tdur), Divide3/2, Divide/2, If Action Subsystem1/2(tdur), If Action Subsystem2/2(tdur), Divide2/2, Divide1/2
  Divide/1 -> Switch1/2
  Divide1/1 -> Switch2/2
  Divide2/1 -> Switch3/2
  Divide3/1 -> Switch/2

== system Gait_Selector/Gait Selector/Trot Gait - Drive Function/right Front Knee gait ==
  t : Inport
  tdur : Inport  Port=2
  Add : Sum
  Constant : Constant  Value=lMin
  Constant10 : Constant  Value=0
  Constant4 : Constant  Value=0
  Divide : Product  Inputs=*/
  Divide1 : Product  Inputs=*/
  Gain7 : Gain  Gain=-(lMax-lMin)
  If Action Subsystem4 : Subsystem  TreatAsAtomicUnit=on
  Switch5 : Switch  Criteria=u2 > Threshold  Threshold=3/8  SaturateOnIntegerOverflow=off  InputSameDT=off
  Switch6 : Switch  Criteria=u2 > Threshold  Threshold=5/8  SaturateOnIntegerOverflow=off  InputSameDT=off
  Out1 : Outport
  wires:
  If Action Subsystem4/1(Out1) -> Switch5/1
  Switch5/1 -> Switch6/3
  t/1 -> Divide1/1, Divide/1, If Action Subsystem4/1(In1)
  Constant4/1 -> Switch5/3
  Constant10/1 -> Switch6/1
  Switch6/1 -> Gain7/1
  Gain7/1 -> Add/1
  Add/1 -> Out1/1
  Constant/1 -> Add/2
  Divide/1 -> Switch5/2
  tdur/1 -> If Action Subsystem4/2(tdur), Divide1/2, Divide/2
  Divide1/1 -> Switch6/2

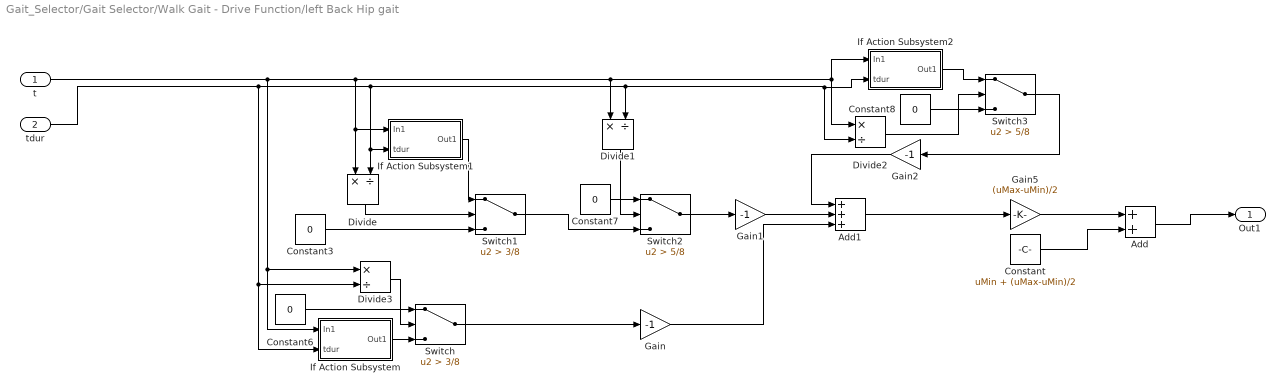
== system Gait_Selector/Gait Selector/Walk Gait - Drive Function/left Back Hip gait ==
  t : Inport
  tdur : Inport  Port=2
  Add : Sum
  Add1 : Sum  Inputs=+++
  Constant : Constant  Value=uMin + (uMax-uMin)/2
  Constant{3,6..8} (4 alike) : Constant  Value=0
  Divide{,1..3} (4 alike) : Product  Inputs=*/
  Gain : Gain  Gain=-1
  Gain1 : Gain  Gain=-1
  Gain2 : Gain  Gain=-1
  Gain5 : Gain  Gain=(uMax-uMin)/2
  If Action Subsystem : Subsystem  TreatAsAtomicUnit=on
  If Action Subsystem1 : Subsystem  TreatAsAtomicUnit=on
  If Action Subsystem2 : Subsystem  TreatAsAtomicUnit=on
  Switch : Switch  Criteria=u2 > Threshold  Threshold=3/8  SaturateOnIntegerOverflow=off  InputSameDT=off
  Switch1 : Switch  Criteria=u2 > Threshold  Threshold=3/8  SaturateOnIntegerOverflow=off  InputSameDT=off
  Switch2 : Switch  Criteria=u2 > Threshold  Threshold=5/8  SaturateOnIntegerOverflow=off  InputSameDT=off
  Switch3 : Switch  Criteria=u2 > Threshold  Threshold=5/8  SaturateOnIntegerOverflow=off  InputSameDT=off
  Out1 : Outport
  wires:
  If Action Subsystem1/1(Out1) -> Switch1/1
  Constant7/1 -> Switch2/1
  Switch1/1 -> Switch2/3
  t/1 -> If Action Subsystem2/1(In1), Divide2/1, Divide1/1, Divide/1, If Action Subsystem1/1(In1), If Action Subsystem/1(In1), Divide3/1
  Add1/1 -> Gain5/1
  If Action Subsystem2/1(Out1) -> Switch3/1
  Switch/1 -> Gain/1
  If Action Subsystem/1(Out1) -> Switch/3
  Constant3/1 -> Switch1/3
  Constant8/1 -> Switch3/3
  Switch3/1 -> Gain2/1
  Switch2/1 -> Gain1/1
  Constant6/1 -> Switch/1
  Gain5/1 -> Add/1
  Constant/1 -> Add/2
  Add/1 -> Out1/1
  Gain/1 -> Add1/3
  Gain1/1 -> Add1/2
  Gain2/1 -> Add1/1
  tdur/1 -> If Action Subsystem/2(tdur), Divide3/2, Divide/2, If Action Subsystem1/2(tdur), If Action Subsystem2/2(tdur), Divide2/2, Divide1/2
  Divide/1 -> Switch1/2
  Divide1/1 -> Switch2/2
  Divide2/1 -> Switch3/2
  Divide3/1 -> Switch/2

== system Gait_Selector/Gait Selector/Walk Gait - Drive Function/left Back Knee gait ==
  t : Inport
  tdur : Inport  Port=2
  Add : Sum
  Constant : Constant  Value=lMin
  Constant10 : Constant  Value=0
  Constant4 : Constant  Value=0
  Divide : Product  Inputs=*/
  Divide1 : Product  Inputs=*/
  Gain7 : Gain  Gain=-(lMax-lMin)
  If Action Subsystem4 : Subsystem  TreatAsAtomicUnit=on
  Switch5 : Switch  Criteria=u2 > Threshold  Threshold=3/8  SaturateOnIntegerOverflow=off  InputSameDT=off
  Switch6 : Switch  Criteria=u2 > Threshold  Threshold=5/8  SaturateOnIntegerOverflow=off  InputSameDT=off
  Out1 : Outport
  wires:
  If Action Subsystem4/1(Out1) -> Switch5/1
  Switch5/1 -> Switch6/3
  t/1 -> Divide1/1, Divide/1, If Action Subsystem4/1(In1)
  Constant4/1 -> Switch5/3
  Constant10/1 -> Switch6/1
  Switch6/1 -> Gain7/1
  Gain7/1 -> Add/1
  Add/1 -> Out1/1
  Constant/1 -> Add/2
  Divide/1 -> Switch5/2
  tdur/1 -> If Action Subsystem4/2(tdur), Divide1/2, Divide/2
  Divide1/1 -> Switch6/2

== system Gait_Selector/Gait Selector/Walk Gait - Drive Function/left Fornt Knee gait ==
  t : Inport
  tdur : Inport  Port=2
  Add : Sum
  Constant : Constant  Value=lMin
  Constant10 : Constant  Value=0
  Constant4 : Constant  Value=0
  Divide : Product  Inputs=*/
  Divide1 : Product  Inputs=*/
  Gain7 : Gain  Gain=-(lMax-lMin)
  If Action Subsystem4 : Subsystem  TreatAsAtomicUnit=on
  Switch5 : Switch  Criteria=u2 > Threshold  Threshold=3/8  SaturateOnIntegerOverflow=off  InputSameDT=off
  Switch6 : Switch  Criteria=u2 > Threshold  Threshold=5/8  SaturateOnIntegerOverflow=off  InputSameDT=off
  Out1 : Outport
  wires:
  If Action Subsystem4/1(Out1) -> Switch5/1
  Switch5/1 -> Switch6/3
  t/1 -> Divide1/1, Divide/1, If Action Subsystem4/1(In1)
  Constant4/1 -> Switch5/3
  Constant10/1 -> Switch6/1
  Switch6/1 -> Gain7/1
  Gain7/1 -> Add/1
  Add/1 -> Out1/1
  Constant/1 -> Add/2
  Divide/1 -> Switch5/2
  tdur/1 -> If Action Subsystem4/2(tdur), Divide1/2, Divide/2
  Divide1/1 -> Switch6/2

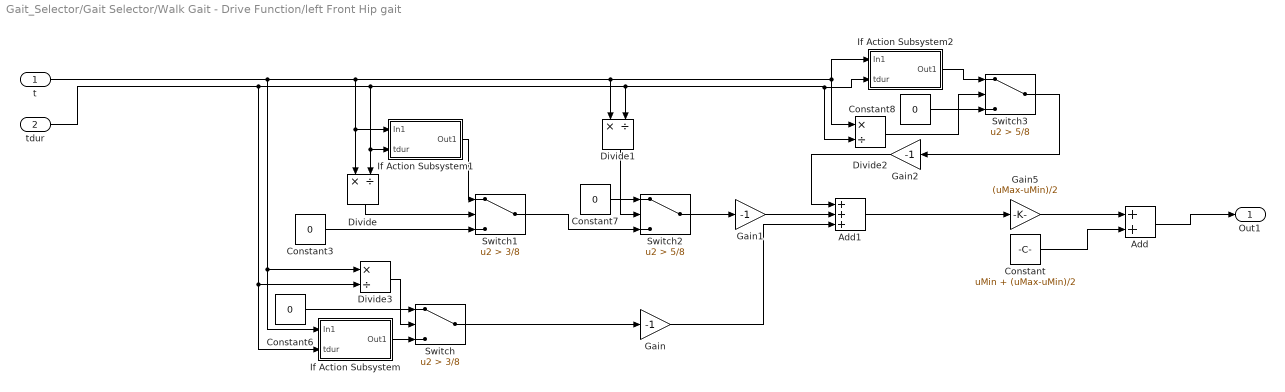
== system Gait_Selector/Gait Selector/Walk Gait - Drive Function/left Front Hip gait ==
  t : Inport
  tdur : Inport  Port=2
  Add : Sum
  Add1 : Sum  Inputs=+++
  Constant : Constant  Value=uMin + (uMax-uMin)/2
  Constant{3,6..8} (4 alike) : Constant  Value=0
  Divide{,1..3} (4 alike) : Product  Inputs=*/
  Gain : Gain  Gain=-1
  Gain1 : Gain  Gain=-1
  Gain2 : Gain  Gain=-1
  Gain5 : Gain  Gain=(uMax-uMin)/2
  If Action Subsystem : Subsystem  TreatAsAtomicUnit=on
  If Action Subsystem1 : Subsystem  TreatAsAtomicUnit=on
  If Action Subsystem2 : Subsystem  TreatAsAtomicUnit=on
  Switch : Switch  Criteria=u2 > Threshold  Threshold=3/8  SaturateOnIntegerOverflow=off  InputSameDT=off
  Switch1 : Switch  Criteria=u2 > Threshold  Threshold=3/8  SaturateOnIntegerOverflow=off  InputSameDT=off
  Switch2 : Switch  Criteria=u2 > Threshold  Threshold=5/8  SaturateOnIntegerOverflow=off  InputSameDT=off
  Switch3 : Switch  Criteria=u2 > Threshold  Threshold=5/8  SaturateOnIntegerOverflow=off  InputSameDT=off
  Out1 : Outport
  wires:
  If Action Subsystem1/1(Out1) -> Switch1/1
  Constant7/1 -> Switch2/1
  Switch1/1 -> Switch2/3
  t/1 -> If Action Subsystem2/1(In1), Divide2/1, Divide1/1, Divide/1, If Action Subsystem1/1(In1), If Action Subsystem/1(In1), Divide3/1
  Add1/1 -> Gain5/1
  If Action Subsystem2/1(Out1) -> Switch3/1
  Switch/1 -> Gain/1
  If Action Subsystem/1(Out1) -> Switch/3
  Constant3/1 -> Switch1/3
  Constant8/1 -> Switch3/3
  Switch3/1 -> Gain2/1
  Switch2/1 -> Gain1/1
  Constant6/1 -> Switch/1
  Gain5/1 -> Add/1
  Constant/1 -> Add/2
  Add/1 -> Out1/1
  Gain/1 -> Add1/3
  Gain1/1 -> Add1/2
  Gain2/1 -> Add1/1
  tdur/1 -> If Action Subsystem/2(tdur), Divide3/2, Divide/2, If Action Subsystem1/2(tdur), If Action Subsystem2/2(tdur), Divide2/2, Divide1/2
  Divide/1 -> Switch1/2
  Divide1/1 -> Switch2/2
  Divide2/1 -> Switch3/2
  Divide3/1 -> Switch/2

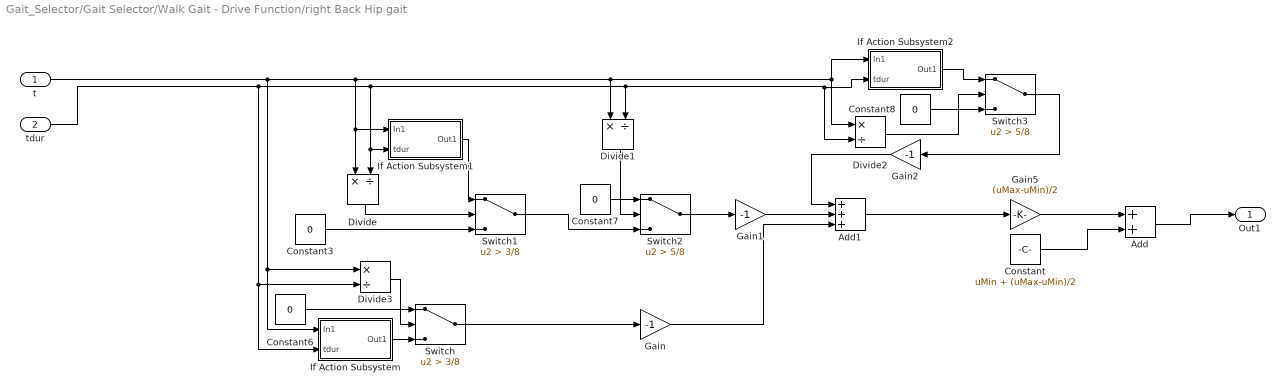
== system Gait_Selector/Gait Selector/Walk Gait - Drive Function/right Back Hip gait ==
  t : Inport
  tdur : Inport  Port=2
  Add : Sum
  Add1 : Sum  Inputs=+++
  Constant : Constant  Value=uMin + (uMax-uMin)/2
  Constant{3,6..8} (4 alike) : Constant  Value=0
  Divide{,1..3} (4 alike) : Product  Inputs=*/
  Gain : Gain  Gain=-1
  Gain1 : Gain  Gain=-1
  Gain2 : Gain  Gain=-1
  Gain5 : Gain  Gain=(uMax-uMin)/2
  If Action Subsystem : Subsystem  TreatAsAtomicUnit=on
  If Action Subsystem1 : Subsystem  TreatAsAtomicUnit=on
  If Action Subsystem2 : Subsystem  TreatAsAtomicUnit=on
  Switch : Switch  Criteria=u2 > Threshold  Threshold=3/8  SaturateOnIntegerOverflow=off  InputSameDT=off
  Switch1 : Switch  Criteria=u2 > Threshold  Threshold=3/8  SaturateOnIntegerOverflow=off  InputSameDT=off
  Switch2 : Switch  Criteria=u2 > Threshold  Threshold=5/8  SaturateOnIntegerOverflow=off  InputSameDT=off
  Switch3 : Switch  Criteria=u2 > Threshold  Threshold=5/8  SaturateOnIntegerOverflow=off  InputSameDT=off
  Out1 : Outport
  wires:
  If Action Subsystem1/1(Out1) -> Switch1/1
  Constant7/1 -> Switch2/1
  Switch1/1 -> Switch2/3
  t/1 -> If Action Subsystem2/1(In1), Divide2/1, Divide1/1, Divide/1, If Action Subsystem1/1(In1), If Action Subsystem/1(In1), Divide3/1
  Add1/1 -> Gain5/1
  If Action Subsystem2/1(Out1) -> Switch3/1
  Switch/1 -> Gain/1
  If Action Subsystem/1(Out1) -> Switch/3
  Constant3/1 -> Switch1/3
  Constant8/1 -> Switch3/3
  Switch3/1 -> Gain2/1
  Switch2/1 -> Gain1/1
  Constant6/1 -> Switch/1
  Gain5/1 -> Add/1
  Constant/1 -> Add/2
  Add/1 -> Out1/1
  Gain/1 -> Add1/3
  Gain1/1 -> Add1/2
  Gain2/1 -> Add1/1
  tdur/1 -> If Action Subsystem/2(tdur), Divide3/2, Divide/2, If Action Subsystem1/2(tdur), If Action Subsystem2/2(tdur), Divide2/2, Divide1/2
  Divide/1 -> Switch1/2
  Divide1/1 -> Switch2/2
  Divide2/1 -> Switch3/2
  Divide3/1 -> Switch/2

== system Gait_Selector/Gait Selector/Walk Gait - Drive Function/right Back Knee gait ==
  t : Inport
  tdur : Inport  Port=2
  Add : Sum
  Constant : Constant  Value=lMin
  Constant10 : Constant  Value=0
  Constant4 : Constant  Value=0
  Divide : Product  Inputs=*/
  Divide1 : Product  Inputs=*/
  Gain7 : Gain  Gain=-(lMax-lMin)
  If Action Subsystem4 : Subsystem  TreatAsAtomicUnit=on
  Switch5 : Switch  Criteria=u2 > Threshold  Threshold=3/8  SaturateOnIntegerOverflow=off  InputSameDT=off
  Switch6 : Switch  Criteria=u2 > Threshold  Threshold=5/8  SaturateOnIntegerOverflow=off  InputSameDT=off
  Out1 : Outport
  wires:
  If Action Subsystem4/1(Out1) -> Switch5/1
  Switch5/1 -> Switch6/3
  t/1 -> Divide1/1, Divide/1, If Action Subsystem4/1(In1)
  Constant4/1 -> Switch5/3
  Constant10/1 -> Switch6/1
  Switch6/1 -> Gain7/1
  Gain7/1 -> Add/1
  Add/1 -> Out1/1
  Constant/1 -> Add/2
  Divide/1 -> Switch5/2
  tdur/1 -> If Action Subsystem4/2(tdur), Divide1/2, Divide/2
  Divide1/1 -> Switch6/2

== system Gait_Selector/Gait Selector/Walk Gait - Drive Function/right Front Hip gait ==
  t : Inport
  tdur : Inport  Port=2
  Add : Sum
  Add1 : Sum  Inputs=+++
  Constant : Constant  Value=uMin + (uMax-uMin)/2
  Constant{3,6..8} (4 alike) : Constant  Value=0
  Divide{,1..3} (4 alike) : Product  Inputs=*/
  Gain : Gain  Gain=-1
  Gain1 : Gain  Gain=-1
  Gain2 : Gain  Gain=-1
  Gain5 : Gain  Gain=(uMax-uMin)/2
  If Action Subsystem : Subsystem  TreatAsAtomicUnit=on
  If Action Subsystem1 : Subsystem  TreatAsAtomicUnit=on
  If Action Subsystem2 : Subsystem  TreatAsAtomicUnit=on
  Switch : Switch  Criteria=u2 > Threshold  Threshold=3/8  SaturateOnIntegerOverflow=off  InputSameDT=off
  Switch1 : Switch  Criteria=u2 > Threshold  Threshold=3/8  SaturateOnIntegerOverflow=off  InputSameDT=off
  Switch2 : Switch  Criteria=u2 > Threshold  Threshold=5/8  SaturateOnIntegerOverflow=off  InputSameDT=off
  Switch3 : Switch  Criteria=u2 > Threshold  Threshold=5/8  SaturateOnIntegerOverflow=off  InputSameDT=off
  Out1 : Outport
  wires:
  If Action Subsystem1/1(Out1) -> Switch1/1
  Constant7/1 -> Switch2/1
  Switch1/1 -> Switch2/3
  t/1 -> If Action Subsystem2/1(In1), Divide2/1, Divide1/1, Divide/1, If Action Subsystem1/1(In1), If Action Subsystem/1(In1), Divide3/1
  Add1/1 -> Gain5/1
  If Action Subsystem2/1(Out1) -> Switch3/1
  Switch/1 -> Gain/1
  If Action Subsystem/1(Out1) -> Switch/3
  Constant3/1 -> Switch1/3
  Constant8/1 -> Switch3/3
  Switch3/1 -> Gain2/1
  Switch2/1 -> Gain1/1
  Constant6/1 -> Switch/1
  Gain5/1 -> Add/1
  Constant/1 -> Add/2
  Add/1 -> Out1/1
  Gain/1 -> Add1/3
  Gain1/1 -> Add1/2
  Gain2/1 -> Add1/1
  tdur/1 -> If Action Subsystem/2(tdur), Divide3/2, Divide/2, If Action Subsystem1/2(tdur), If Action Subsystem2/2(tdur), Divide2/2, Divide1/2
  Divide/1 -> Switch1/2
  Divide1/1 -> Switch2/2
  Divide2/1 -> Switch3/2
  Divide3/1 -> Switch/2

== system Gait_Selector/Gait Selector/Walk Gait - Drive Function/right Front Knee gait ==
  t : Inport
  tdur : Inport  Port=2
  Add : Sum
  Constant : Constant  Value=lMin
  Constant10 : Constant  Value=0
  Constant4 : Constant  Value=0
  Divide : Product  Inputs=*/
  Divide1 : Product  Inputs=*/
  Gain7 : Gain  Gain=-(lMax-lMin)
  If Action Subsystem4 : Subsystem  TreatAsAtomicUnit=on
  Switch5 : Switch  Criteria=u2 > Threshold  Threshold=3/8  SaturateOnIntegerOverflow=off  InputSameDT=off
  Switch6 : Switch  Criteria=u2 > Threshold  Threshold=5/8  SaturateOnIntegerOverflow=off  InputSameDT=off
  Out1 : Outport
  wires:
  If Action Subsystem4/1(Out1) -> Switch5/1
  Switch5/1 -> Switch6/3
  t/1 -> Divide1/1, Divide/1, If Action Subsystem4/1(In1)
  Constant4/1 -> Switch5/3
  Constant10/1 -> Switch6/1
  Switch6/1 -> Gain7/1
  Gain7/1 -> Add/1
  Add/1 -> Out1/1
  Constant/1 -> Add/2
  Divide/1 -> Switch5/2
  tdur/1 -> If Action Subsystem4/2(tdur), Divide1/2, Divide/2
  Divide1/1 -> Switch6/2

== system Gait_Selector/Gait Selector/Trot Gait - Drive Function/left Back Hip gait/If Action Subsystem ==
  In1 : Inport
  tdur : Inport  Port=2
  Add : Sum  Inputs=+-
  Constant : Constant  Value=1.5 * pi
  Divide : Product  Inputs=*/
  Gain1 : Gain  Gain=2/3
  Gain4 : Gain  Gain=2*pi
  Sin : Trigonometry
  Out1 : Outport
  wires:
  In1/1 -> Gain4/1
  Constant/1 -> Add/2
  Add/1 -> Gain1/1
  Gain1/1 -> Sin/1
  Sin/1 -> Out1/1
  Gain4/1 -> Divide/1
  tdur/1 -> Divide/2
  Divide/1 -> Add/1

== system Gait_Selector/Gait Selector/Trot Gait - Drive Function/left Back Hip gait/If Action Subsystem1 ==
  In1 : Inport
  tdur : Inport  Port=2
  Add : Sum  Inputs=+-
  Constant : Constant  Value=1.0 * pi
  Divide : Product  Inputs=*/
  Gain1 : Gain  Gain=2
  Gain4 : Gain  Gain=2*pi
  Sin : Trigonometry
  Out1 : Outport
  wires:
  Sin/1 -> Out1/1
  In1/1 -> Gain4/1
  Add/1 -> Gain1/1
  Constant/1 -> Add/2
  Gain1/1 -> Sin/1
  Gain4/1 -> Divide/1
  Divide/1 -> Add/1
  tdur/1 -> Divide/2

== system Gait_Selector/Gait Selector/Trot Gait - Drive Function/left Back Hip gait/If Action Subsystem2 ==
  In1 : Inport
  tdur : Inport  Port=2
  Add : Sum  Inputs=+-
  Constant : Constant  Value=1.25 * pi
  Divide : Product  Inputs=*/
  Gain1 : Gain  Gain=2/3
  Gain4 : Gain  Gain=2*pi
  Sin : Trigonometry  Operator=cos
  Out1 : Outport
  wires:
  Sin/1 -> Out1/1
  In1/1 -> Gain4/1
  Add/1 -> Gain1/1
  Constant/1 -> Add/2
  Gain1/1 -> Sin/1
  Gain4/1 -> Divide/1
  Divide/1 -> Add/1
  tdur/1 -> Divide/2

== system Gait_Selector/Gait Selector/Trot Gait - Drive Function/left Back Knee gait/If Action Subsystem4 ==
  In1 : Inport
  tdur : Inport  Port=2
  Add : Sum  Inputs=+-
  Constant : Constant  Value=0.75 * pi
  Divide : Product  Inputs=*/
  Gain1 : Gain  Gain=2
  Gain4 : Gain  Gain=2*pi
  Sin : Trigonometry
  Out1 : Outport
  wires:
  Sin/1 -> Out1/1
  In1/1 -> Gain4/1
  Add/1 -> Gain1/1
  Constant/1 -> Add/2
  Gain1/1 -> Sin/1
  Divide/1 -> Add/1
  Gain4/1 -> Divide/1
  tdur/1 -> Divide/2

== system Gait_Selector/Gait Selector/Trot Gait - Drive Function/left Front Hip gait/If Action Subsystem ==
  In1 : Inport
  tdur : Inport  Port=2
  Add : Sum  Inputs=+-
  Constant : Constant  Value=1.5 * pi
  Divide : Product  Inputs=*/
  Gain1 : Gain  Gain=2/3
  Gain4 : Gain  Gain=2*pi
  Sin : Trigonometry
  Out1 : Outport
  wires:
  In1/1 -> Gain4/1
  Constant/1 -> Add/2
  Add/1 -> Gain1/1
  Gain1/1 -> Sin/1
  Sin/1 -> Out1/1
  Gain4/1 -> Divide/1
  tdur/1 -> Divide/2
  Divide/1 -> Add/1

== system Gait_Selector/Gait Selector/Trot Gait - Drive Function/left Front Hip gait/If Action Subsystem1 ==
  In1 : Inport
  tdur : Inport  Port=2
  Add : Sum  Inputs=+-
  Constant : Constant  Value=1.0 * pi
  Divide : Product  Inputs=*/
  Gain1 : Gain  Gain=2
  Gain4 : Gain  Gain=2*pi
  Sin : Trigonometry
  Out1 : Outport
  wires:
  Sin/1 -> Out1/1
  In1/1 -> Gain4/1
  Add/1 -> Gain1/1
  Constant/1 -> Add/2
  Gain1/1 -> Sin/1
  Gain4/1 -> Divide/1
  Divide/1 -> Add/1
  tdur/1 -> Divide/2

== system Gait_Selector/Gait Selector/Trot Gait - Drive Function/left Front Hip gait/If Action Subsystem2 ==
  In1 : Inport
  tdur : Inport  Port=2
  Add : Sum  Inputs=+-
  Constant : Constant  Value=1.25 * pi
  Divide : Product  Inputs=*/
  Gain1 : Gain  Gain=2/3
  Gain4 : Gain  Gain=2*pi
  Sin : Trigonometry  Operator=cos
  Out1 : Outport
  wires:
  Sin/1 -> Out1/1
  In1/1 -> Gain4/1
  Add/1 -> Gain1/1
  Constant/1 -> Add/2
  Gain1/1 -> Sin/1
  Gain4/1 -> Divide/1
  Divide/1 -> Add/1
  tdur/1 -> Divide/2

== system Gait_Selector/Gait Selector/Trot Gait - Drive Function/left Front Knee gait/If Action Subsystem4 ==
  In1 : Inport
  tdur : Inport  Port=2
  Add : Sum  Inputs=+-
  Constant : Constant  Value=0.75 * pi
  Divide : Product  Inputs=*/
  Gain1 : Gain  Gain=2
  Gain4 : Gain  Gain=2*pi
  Sin : Trigonometry
  Out1 : Outport
  wires:
  Sin/1 -> Out1/1
  In1/1 -> Gain4/1
  Add/1 -> Gain1/1
  Constant/1 -> Add/2
  Gain1/1 -> Sin/1
  Divide/1 -> Add/1
  Gain4/1 -> Divide/1
  tdur/1 -> Divide/2
